simulink model "HXpump_whole"  (R2014b)
settings: Solver=FixedStepDiscrete  StartTime=0.0  StopTime=Tfinal  FixedStep=Ts  RelTol=1e-3
values from neighbouring files (symbols this model uses):
  A = wallpar(4)    [EKFdynamics.m]    (also in heatexchanger.m; heatexchangerpump.m; hxpumpcode.m = params.A; hxpumpcodesanity.m = 292.2)
  cc = coldpar(3)    [EKFdynamics.m]    (also in heatexchanger.m; heatexchangerpump.m; hxpumpcode.m = params.cc; hxpumpcodesanity.m = 1901)
  ch = hotpar(3)    [EKFdynamics.m]    (also in heatexchanger.m; heatexchangerpump.m; hxpumpcode.m = params.ch; hxpumpcodesanity.m = 2414)
  cw = wallpar(3)    [EKFdynamics.m]    (also in heatexchanger.m; heatexchangerpump.m; hxpumpcode.m = params.cw; hxpumpcodesanity.m = 578)
  filenameAsnum = uint8(filename)    [hxpumpcode.m]
  h = params.Ts    [hxpumpcode.m]    (also in hxpumpcodesanity.m = 0.1; noErrornoDelay.mat = 0.1)
  hc = coldpar(4)    [EKFdynamics.m]    (also in heatexchanger.m; heatexchangerpump.m; hxpumpcode.m = params.hc; hxpumpcodesanity.m = 24500)
  hh = hotpar(5)    [EKFdynamics.m]    (also in heatexchanger.m; heatexchangerpump.m; hxpumpcode.m = params.hh; hxpumpcodesanity.m = 23800)
  ki = 1.2    [HeatExchanger_ps.m]    (also in hxpumpcode.m = 1; hxpumpcodesanity.m; noErrornoDelay.mat = 1)
  kp = 4.995    [HeatExchanger_ps.m]    (also in hxpumpcode.m = 4; hxpumpcodesanity.m; noErrornoDelay.mat = 4)
  mdotc = input(1)    [EKFdynamics.m]    (also in heatexchanger.m; heatexchangerpump.m; hxpumpcode.m = 210.8; hxpumpcodesanity.m = 247)
  mdoth = hotpar(4)    [EKFdynamics.m]    (also in heatexchanger.m; heatexchangerpump.m; hxpumpcode.m = params.mdoth; hxpumpcodesanity.m = 350)
  PDT = [0.0475545264184 0.219864503106 0.124236222348 0.000344859251401 0.00269336621478 0 0.219864503106 2.46009324019 0.934080700726 -7.94146801374e-05 -0.000620231546177 0 ... (36 elements, 6x6)]    [noErrornoDelay.mat]
  Pref = params.Pref    [hxpumpcode.m]    (also in hxpumpcodesanity.m = 37.8; noErrornoDelay.mat = 37.8)
  rhoc = coldpar(1)    [EKFdynamics.m]    (also in heatexchanger.m; heatexchangerpump.m; hxpumpcode.m = params.rhoc; hxpumpcodesanity.m = 2020)
  rhoh = hotpar(1)    [EKFdynamics.m]    (also in heatexchanger.m; heatexchangerpump.m; hxpumpcode.m = params.rhoh; hxpumpcodesanity.m = 1940)
  rhow = wallpar(1)    [EKFdynamics.m]    (also in heatexchanger.m; heatexchangerpump.m; hxpumpcode.m = params.rhow; hxpumpcodesanity.m = 8860)
  Sv_mh = 0.05    [HeatExchanger_ps.m]    (also in hxpumpcode.m = params.Sv_mh; hxpumpcodesanity.m; noErrornoDelay.mat)
  Sv_thi = 5e-2    (= 0.05)    [HeatExchanger_ps.m]    (also in hxpumpcode.m = params.Sv_thi; hxpumpcodesanity.m; noErrornoDelay.mat)
  Sv_tho = 0.1    [HeatExchanger_ps.m]    (also in hxpumpcode.m = params.Sv_tho; hxpumpcodesanity.m; noErrornoDelay.mat)
  Sw_mh = 25    [HeatExchanger_ps.m]    (also in hxpumpcode.m = params.Sw_mh; hxpumpcodesanity.m; noErrornoDelay.mat)
  Sw_tc = 0.05    [HeatExchanger_ps.m]    (also in hxpumpcode.m = params.Sw_tc; hxpumpcodesanity.m; noErrornoDelay.mat)
  Sw_th = 25    [HeatExchanger_ps.m]    (also in hxpumpcode.m = params.Sw_th; hxpumpcodesanity.m; noErrornoDelay.mat)
  Tci = input(2)    [EKFdynamics.m]    (also in heatexchanger.m; heatexchangerpump.m; hxpumpcode.m = params.Tci; hxpumpcodesanity.m = 550)
  Thi = hotpar(6)    [EKFdynamics.m]    (also in heatexchanger.m; heatexchangerpump.m; hxpumpcode.m = params.Thi; hxpumpcodesanity.m = 700)
  Ts = delta_t    (= 0.1)    [HeatExchanger_ps.m]    (also in hxpumpcode.m = params.Ts; hxpumpcodesanity.m; noErrornoDelay.mat)
  Vc = coldpar(2)    [EKFdynamics.m]    (also in heatexchanger.m; heatexchangerpump.m; hxpumpcode.m = params.Vc; hxpumpcodesanity.m = 1.5127)
  Vh = hotpar(2)    [EKFdynamics.m]    (also in heatexchanger.m; heatexchangerpump.m; hxpumpcode.m = params.Vh; hxpumpcodesanity.m = 1.1508)
  Vw = wallpar(2)    [EKFdynamics.m]    (also in heatexchanger.m; heatexchangerpump.m; hxpumpcode.m = params.Vw; hxpumpcodesanity.m = 0.4675)
  wa = pumppar(2)    [EKFdynamics.m]    (also in hxpumpcode.m = params.wa; hxpumpcodesanity.m = 0.002; noErrornoDelay.mat = 0.002)
  wb = pumppar(3)    [EKFdynamics.m]    (also in hxpumpcode.m = params.wb; hxpumpcodesanity.m = 0.005; noErrornoDelay.mat = 0.005)
  wp = pumppar(1)    [EKFdynamics.m]    (also in heatexchangerpump.m; hxpumpcode.m = params.wp; hxpumpcodesanity.m = 0.1; noErrornoDelay.mat = 0.1)
  wref = params.wref    [hxpumpcode.m]    (also in hxpumpcodesanity.m = 0.1; noErrornoDelay.mat = 0.1)
  x0 = tempx0'    [hxpumpcode.m]    (also in hxpumpcodesanity.m = [650.29 638.4 644.3 mdoth Thi 250]; noErrornoDelay.mat = [655.2 644.46 649.75 350 700 210.8])
libraries: simulink x6, powerlib_meascontrol x3
settings Model: Creator=LabUser  LastModifiedBy=sc16user
settings DataIOCC: LimitDataPoints=off  SignalLoggingSaveFormat=ModelDataLogs
settings DebuggingCC: UnderspecifiedInitializationDetection=Classic  MergeDetectMultiDrivingBlocksExec=none  MultiTaskDSMMsg=warning  MultiTaskCondExecSysMsg=none  StateNameClashWarn=warning
settings RTWCC: IncludeERTFirstTime=on

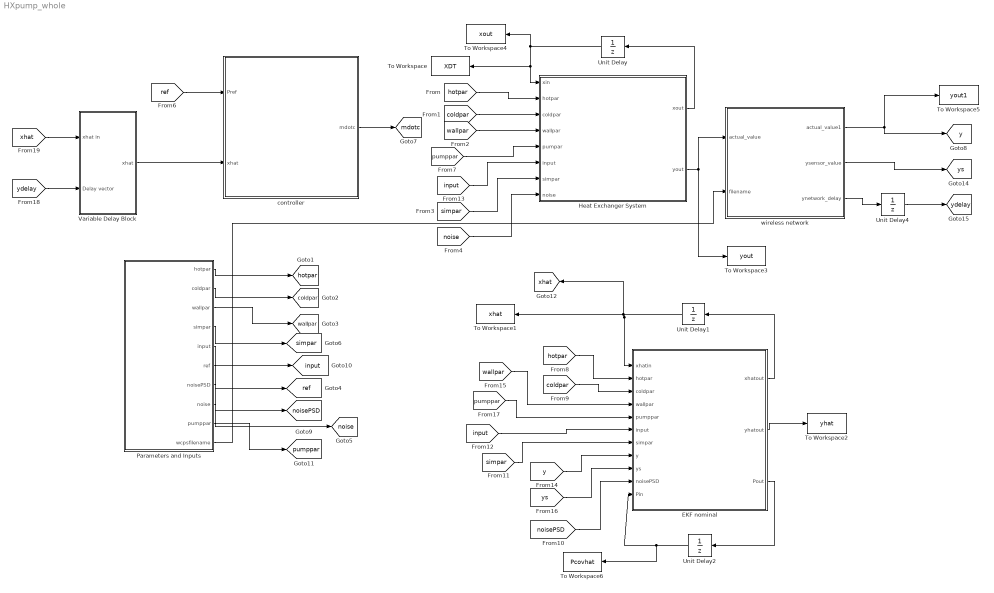
== system HXpump_whole ==
  EKF nominal : MATLAB Function  TreatAsAtomicUnit=on
  Heat Exchanger System : MATLAB Function  TreatAsAtomicUnit=on
  Parameters and Inputs : Subsystem
  To Workspace : ToWorkspace  VariableName=XDT  SampleTime=-1
  To Workspace1 : ToWorkspace  VariableName=xhat  SampleTime=-1
  To Workspace2 : ToWorkspace  VariableName=yhat  SampleTime=-1
  To Workspace3 : ToWorkspace  VariableName=yout  SampleTime=-1
  To Workspace4 : ToWorkspace  VariableName=xout  SampleTime=-1
  To Workspace5 : ToWorkspace  VariableName=yout1  SampleTime=-1
  To Workspace6 : ToWorkspace  VariableName=Pcovhat  SampleTime=-1
  Unit Delay : UnitDelay  InitialCondition=x0([1 2 3 6])  SampleTime=-1
  Unit Delay1 : UnitDelay  InitialCondition=x0  SampleTime=-1
  Unit Delay2 : UnitDelay  InitialCondition=PDT  SampleTime=-1
  Unit Delay4 : UnitDelay  InitialCondition=[0 0 0]  SampleTime=-1
  Variable Delay Block : Subsystem
  controller : Subsystem
  wireless network : MATLAB Function  TreatAsAtomicUnit=on  SystemSampleTime=0.1
  tag scope: coldpar=global, hotpar=global, input=global, mdotc=global, noise=global, noisePSD=global, pumppar=global, ref=global, simpar=global, wallpar=global, xhat=global, y=global, ydelay=global, ys=global
  wires:
  Unit Delay/1 -> To Workspace4/1, To Workspace/1, Heat Exchanger System/1(xin)
  Heat Exchanger System/1(xout) -> Unit Delay/1
  [hotpar] -> Heat Exchanger System/2(hotpar)
  [coldpar] -> Heat Exchanger System/3(coldpar)
  [wallpar] -> Heat Exchanger System/4(wallpar)
  [simpar] -> Heat Exchanger System/7(simpar)
  [noise] -> Heat Exchanger System/8(noise)
  [input] -> Heat Exchanger System/6(input)
  [ref] -> controller/1(Pref)
  Variable Delay Block/1(xhat) -> controller/2(xhat)
  controller/1(mdotc) -> [mdotc]
  [pumppar] -> Heat Exchanger System/5(pumpar)
  Parameters and Inputs/1(hotpar) -> [hotpar]
  Parameters and Inputs/2(coldpar) -> [coldpar]
  Parameters and Inputs/3(wallpar) -> [wallpar]
  Parameters and Inputs/4(simpar) -> [simpar]
  Parameters and Inputs/5(input) -> [input]
  Parameters and Inputs/6(ref) -> [ref]
  Parameters and Inputs/8(noise) -> [noise]
  Parameters and Inputs/7(noisePSD) -> [noisePSD]
  Parameters and Inputs/9(pumppar) -> [pumppar]
  [hotpar] -> EKF nominal/2(hotpar)
  [coldpar] -> EKF nominal/3(coldpar)
  [wallpar] -> EKF nominal/4(wallpar)
  [simpar] -> EKF nominal/7(simpar)
  [y] -> EKF nominal/8(y)
  [noisePSD] -> EKF nominal/10(noisePSD)
  Unit Delay1/1 -> EKF nominal/1(xhatin), To Workspace1/1, [xhat]
  EKF nominal/1(xhatout) -> Unit Delay1/1
  EKF nominal/3(Pout) -> Unit Delay2/1
  Unit Delay2/1 -> To Workspace6/1, EKF nominal/11(Pin)
  EKF nominal/2(yhatout) -> To Workspace2/1
  [input] -> EKF nominal/6(input)
  [ys] -> EKF nominal/9(ys)
  [pumppar] -> EKF nominal/5(pumppar)
  wireless network/1(actual_value1) -> [y], To Workspace5/1
  wireless network/2(ysensor_value) -> [ys]
  wireless network/3(ynetwork_delay) -> Unit Delay4/1
  Unit Delay4/1 -> [ydelay]
  Heat Exchanger System/2(yout) -> To Workspace3/1, wireless network/1(actual_value)
  [xhat] -> Variable Delay Block/1(xhat in)
  [ydelay] -> Variable Delay Block/2(Delay vector)
  Parameters and Inputs/10(wcpsfilename) -> wireless network/2(filename)

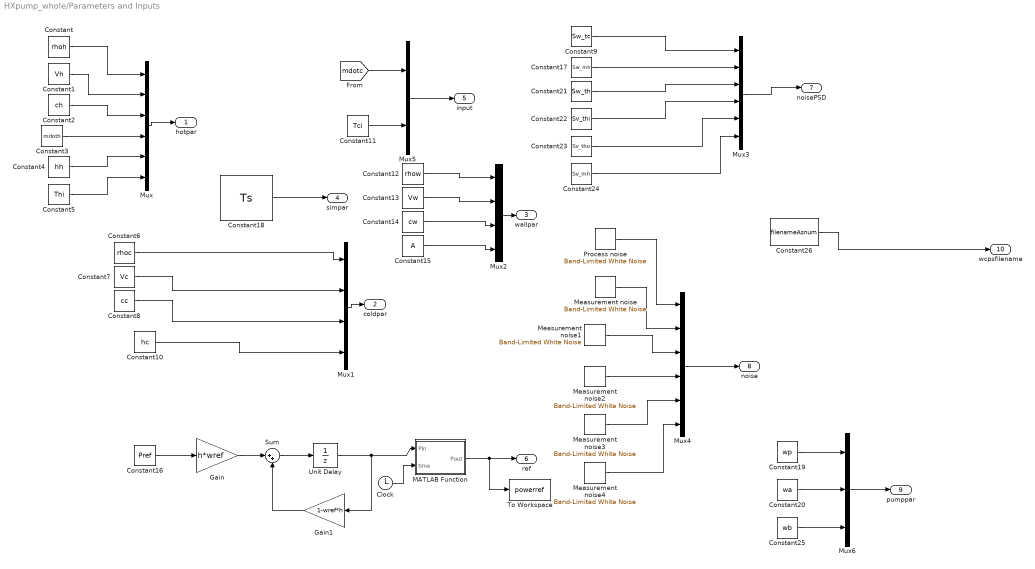
== system HXpump_whole/Parameters and Inputs ==
  Clock : Clock
  Constant : Constant  Value=rhoh  SampleTime=Ts
  Constant1 : Constant  Value=Vh  SampleTime=Ts
  Constant10 : Constant  Value=hc  SampleTime=Ts
  Constant11 : Constant  Value=Tci  SampleTime=Ts
  Constant12 : Constant  Value=rhow  SampleTime=Ts
  Constant13 : Constant  Value=Vw  SampleTime=Ts
  Constant14 : Constant  Value=cw  SampleTime=Ts
  Constant15 : Constant  Value=A  SampleTime=Ts
  Constant16 : Constant  Value=Pref  SampleTime=Ts
  Constant17 : Constant  Value=Sw_mh  SampleTime=Ts
  Constant18 : Constant  Value=Ts  SampleTime=Ts
  Constant19 : Constant  Value=wp  SampleTime=Ts
  Constant2 : Constant  Value=ch  SampleTime=Ts
  Constant20 : Constant  Value=wa  SampleTime=Ts
  Constant21 : Constant  Value=Sw_th  SampleTime=Ts
  Constant22 : Constant  Value=Sv_thi  SampleTime=Ts
  Constant23 : Constant  Value=Sv_tho  SampleTime=Ts
  Constant24 : Constant  Value=Sv_mh  SampleTime=Ts
  Constant25 : Constant  Value=wb  SampleTime=Ts
  Constant26 : Constant  Value=filenameAsnum  SampleTime=Ts
  Constant3 : Constant  Value=mdoth  SampleTime=Ts
  Constant4 : Constant  Value=hh  SampleTime=Ts
  Constant5 : Constant  Value=Thi  SampleTime=Ts
  Constant6 : Constant  Value=rhoc  SampleTime=Ts
  Constant7 : Constant  Value=Vc  SampleTime=Ts
  Constant8 : Constant  Value=cc  SampleTime=Ts
  Constant9 : Constant  Value=Sw_tc  SampleTime=Ts
  Gain : Gain  Gain=h*wref
  Gain1 : Gain  Gain=1-wref*h
  MATLAB Function : MATLAB Function  TreatAsAtomicUnit=on
  Measurement noise : simulink/Sources/Band-Limited White Noise  Cov=0  Ts=Ts  seed=[12345]
  Measurement noise1 : simulink/Sources/Band-Limited White Noise  Cov=0  Ts=Ts  seed=[23456]
  Measurement noise2 : simulink/Sources/Band-Limited White Noise  Cov=0*Ts  Ts=Ts  seed=[34567]
  Measurement noise3 : simulink/Sources/Band-Limited White Noise  Cov=0*Ts  Ts=Ts  seed=[45678]
  Measurement noise4 : simulink/Sources/Band-Limited White Noise  Cov=0*Ts  Ts=Ts  seed=[11111]
  Mux : Mux  Inputs=6
  Mux1 : Mux
  Mux2 : Mux
  Mux3 : Mux  Inputs=6
  Mux4 : Mux  Inputs=6
  Mux5 : Mux  Inputs=2
  Mux6 : Mux  Inputs=3
  Process noise : simulink/Sources/Band-Limited White Noise  Cov=0  Ts=Ts  seed=[23341]
  Sum : Sum  Inputs=|++
  To Workspace : ToWorkspace  VariableName=powerref  SampleTime=-1
  Unit Delay : UnitDelay  InitialCondition=Pref  SampleTime=-1
  hotpar : Outport
  coldpar : Outport  Port=2
  wallpar : Outport  Port=3
  simpar : Outport  Port=4
  input : Outport  Port=5
  ref : Outport  Port=6
  noisePSD : Outport  Port=7
  noise : Outport  Port=8
  pumppar : Outport  Port=9
  wcpsfilename : Outport  Port=10
  wires:
  Constant1/1 -> Mux/2
  Constant/1 -> Mux/1
  Mux/1 -> hotpar/1
  Constant2/1 -> Mux/3
  Constant6/1 -> Mux1/1
  Mux1/1 -> coldpar/1
  Constant8/1 -> Mux1/3
  Constant7/1 -> Mux1/2
  Mux2/1 -> wallpar/1
  Constant10/1 -> Mux1/4
  Constant12/1 -> Mux2/1
  Constant13/1 -> Mux2/2
  Constant14/1 -> Mux2/3
  Constant15/1 -> Mux2/4
  Constant18/1 -> simpar/1
  Constant4/1 -> Mux/5
  Mux5/1 -> input/1
  [mdotc] -> Mux5/1
  Constant11/1 -> Mux5/2
  Constant3/1 -> Mux/4
  Constant5/1 -> Mux/6
  Constant17/1 -> Mux3/2
  Constant9/1 -> Mux3/1
  Mux3/1 -> noisePSD/1
  Process noise/1 -> Mux4/1
  Measurement noise/1 -> Mux4/2
  Measurement noise1/1 -> Mux4/3
  Measurement noise2/1 -> Mux4/4
  Measurement noise3/1 -> Mux4/5
  Measurement noise4/1 -> Mux4/6
  Constant21/1 -> Mux3/3
  Constant22/1 -> Mux3/4
  Constant23/1 -> Mux3/5
  Constant24/1 -> Mux3/6
  Mux4/1 -> noise/1
  Constant16/1 -> Gain/1
  Gain/1 -> Sum/1
  Sum/1 -> Unit Delay/1
  Unit Delay/1 -> MATLAB Function/1(Pin), Gain1/1
  Gain1/1 -> Sum/2
  Constant19/1 -> Mux6/1
  Constant20/1 -> Mux6/2
  Constant25/1 -> Mux6/3
  Mux6/1 -> pumppar/1
  Clock/1 -> MATLAB Function/2(time)
  MATLAB Function/1(Pout) -> To Workspace/1, ref/1
  Constant26/1 -> wcpsfilename/1

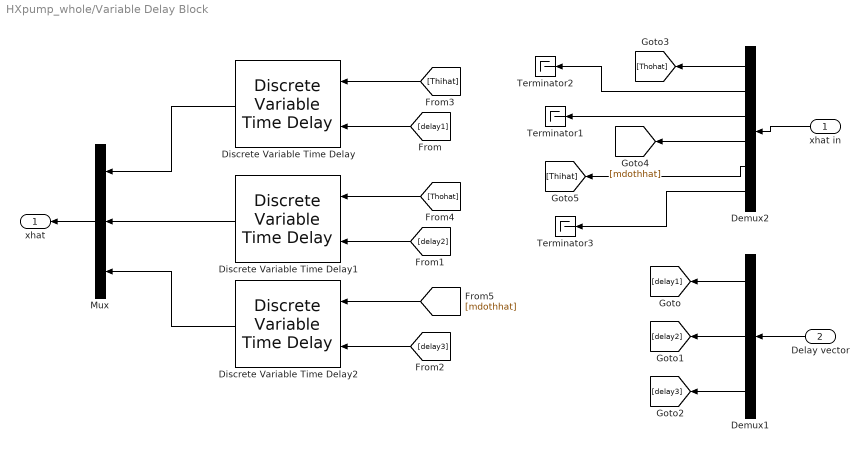
== system HXpump_whole/Variable Delay Block ==
  xhat in : Inport
  Delay vector : Inport  Port=2
  Demux1 : Demux  Outputs=3
  Demux2 : Demux  Outputs=6
  Discrete Variable Time Delay : powerlib_meascontrol/Additional Components/Discrete Variable Time Delay  MaxDelay=2  InitialValue=700  Ts=Ts  DFT=on
  Discrete Variable Time Delay1 : powerlib_meascontrol/Additional Components/Discrete Variable Time Delay  MaxDelay=2  InitialValue=650.29  Ts=Ts  DFT=on
  Discrete Variable Time Delay2 : powerlib_meascontrol/Additional Components/Discrete Variable Time Delay  MaxDelay=2  InitialValue=350  Ts=Ts  DFT=on
  Mux : Mux  Inputs=3
  Terminator1 : Terminator
  Terminator2 : Terminator
  Terminator3 : Terminator
  xhat : Outport
  wires:
  Discrete Variable Time Delay2/1 -> Mux/3
  Discrete Variable Time Delay/1 -> Mux/1
  Delay vector/1 -> Demux1/1
  Discrete Variable Time Delay1/1 -> Mux/2
  Demux1/1 -> [delay1]
  Demux1/2 -> [delay2]
  Demux1/3 -> [delay3]
  [delay1] -> Discrete Variable Time Delay/2
  [delay2] -> Discrete Variable Time Delay1/2
  [delay3] -> Discrete Variable Time Delay2/2
  [Thihat] -> Discrete Variable Time Delay/1
  [Thohat] -> Discrete Variable Time Delay1/1
  [mdothhat] -> Discrete Variable Time Delay2/1
  Mux/1 -> xhat/1
  xhat in/1 -> Demux2/1
  Demux2/1 -> [Thohat]
  Demux2/4 -> [mdothhat]
  Demux2/5 -> [Thihat]
  Demux2/3 -> Terminator1/1
  Demux2/2 -> Terminator2/1
  Demux2/6 -> Terminator3/1

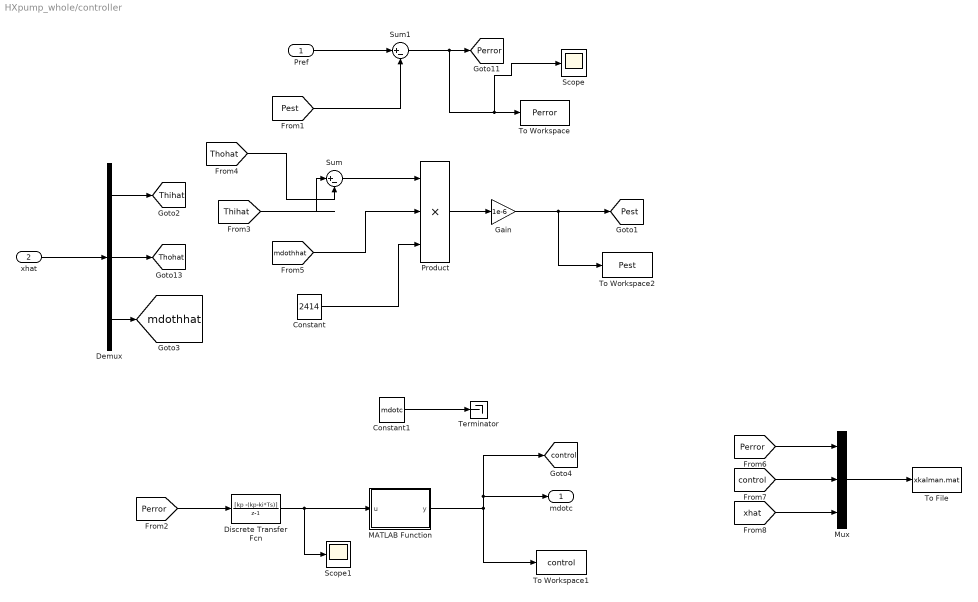
== system HXpump_whole/controller ==
  Pref : Inport
  xhat : Inport  Port=2
  Constant : Constant  Value=2414  SampleTime=Ts
  Constant1 : Constant  Value=mdotc
  Demux : Demux  Outputs=3
  Discrete Transfer Fcn : DiscreteTransferFcn  Numerator=[kp -(kp-ki*Ts)]  Denominator=[1 -1]  InitialStates=250.6/Ts  SampleTime=Ts
  Gain : Gain  Gain=1e-6
  MATLAB Function : MATLAB Function  TreatAsAtomicUnit=on
  Mux : Mux  Inputs=3
  Product : Product  Inputs=3
  Scope : Scope
  Scope1 : Scope
  Sum : Sum  Inputs=|+-
  Sum1 : Sum  Inputs=|+-
  Terminator : Terminator
  To File : ToFile  Filename=xkalman.mat  MatrixName=xkalman
  To Workspace : ToWorkspace  VariableName=Perror  SampleTime=-1
  To Workspace1 : ToWorkspace  VariableName=control  SampleTime=-1
  To Workspace2 : ToWorkspace  VariableName=Pest  SampleTime=-1
  mdotc : Outport
  tag scope: Perror=global, Pest=global, Thihat=global, Thohat=global, control=global, mdothhat=global
  wires:
  [Thohat] -> Sum/2
  [mdothhat] -> Product/2
  Sum/1 -> Product/1
  Constant/1 -> Product/3
  xhat/1 -> Demux/1
  Product/1 -> Gain/1
  Pref/1 -> Sum1/1
  Gain/1 -> To Workspace2/1, [Pest]
  [Pest] -> Sum1/2
  Sum1/1 -> To Workspace/1, Scope/1, [Perror]
  Discrete Transfer Fcn/1 -> Scope1/1, MATLAB Function/1(u)
  [Perror] -> Discrete Transfer Fcn/1
  [Thihat] -> Sum/1
  Demux/3 -> [mdothhat]
  Demux/2 -> [Thohat]
  Demux/1 -> [Thihat]
  [Perror] -> Mux/1
  [control] -> Mux/2
  Mux/1 -> To File/1
  [xhat] -> Mux/3
  Constant1/1 -> Terminator/1
  MATLAB Function/1(y) -> [control], mdotc/1, To Workspace1/1

== matlab function HXpump_whole/EKF nominal ==
  data: xhatin input; hotpar input; coldpar input; wallpar input; pumppar input; input input; simpar input; y input; ys input; noisePSD input; Pin input; xhatout output; yhatout output; Pout output
function [xhatout,yhatout,Pout] = fcn(xhatin,hotpar,coldpar,wallpar,pumppar,input,simpar,y,ys,noisePSD,Pin)
%#codegen

% simulation parameters
h = simpar(1);

% hot-leg parameters
rhoh  = hotpar(1);
Vh    = hotpar(2);
ch    = hotpar(3);
mdoth = hotpar(4);
hh    = hotpar(5);
Thi   = hotpar(6);

% cold-leg parameters
rhoc  = coldpar(1);
Vc    = coldpar(2);
cc    = coldpar(3);
hc    = coldpar(4);

% inputs
mdotc = input(1);
Tci   = input(2);

% wall parameters
rhow  = wallpar(1);
Vw    = wallpar(2);
cw    = wallpar(3);
A     = wallpar(4);

% pump and disturbance parameters
wp = pumppar(1);
wa = pumppar(2);
wb = pumppar(3);

% noisePSD
Sw_tc  = noisePSD(1);
Sw_mh  = noisePSD(2);
Sw_th  = noisePSD(3);
Sw = diag([Sw_tc Sw_mh Sw_th]);

Sv_thi = noisePSD(4);
Sv_tho = noisePSD(5);
Sv_mh  = noisePSD(6);
Sv = diag([Sv_thi Sv_tho Sv_mh]);

% fourth order Runga Kutta
c1 = 1/6;
c2 = 1/3;
c3 = 1/3;
c4 = 1/6;
a2 = 1/2;
a3 = 1/2;
a4 = 1;
b21 = 1/2;
b31 = 0;
b32 = 1/2;
b41 = 0;
b42 = 0;
b43 = 1;

K1 = EKFdynamics(xhatin,hotpar,coldpar,wallpar,pumppar,input);
K2 = EKFdynamics(xhatin+b21*K1*h,hotpar,coldpar,wallpar,pumppar,input);
K3 = EKFdynamics(xhatin+b31*K1*h+b32*K2*h,hotpar,coldpar,wallpar,pumppar,input);
K4 = EKFdynamics(xhatin+b41*K1*h+b42*K2*h+b43*K3*h,hotpar,coldpar,wallpar,pumppar,input);
slope   = c1*K1+c2*K2+c3*K3+c4*K4;

% State Matrices in Continuous-Time
ACT = [-(xhatin(4)*ch + hh*A)/(rhoh*Vh*ch) 0 hh*A/(rhoh*Vh*ch) ch*(xhatin(5) - xhatin(1))/(rhoh*Vh*ch) xhatin(4)*ch/(rhoh*Vh*ch) 0;
       0 -(mdotc*cc + hc*A)/(rhoc*Vc*cc) hc*A/(rhoc*Vc*cc) 0 0 cc*(Tci-xhatin(2))/(rhoc*Vc*cc);
       hh*A/(rhow*Vw*cw) hc*A/(rhow*Vw*cw) -(hh*A + hc*A)/(rhow*Vw*cw) 0 0 0;
       0 0 0 -wa 0 0;
       0 0 0 0 -wb 0;
       0 0 0 0 0 -wp];
BwCT = [0 0 0  ; mdotc*cc/(rhoc*Vc*cc)*Tci 0 0 ; zeros(1,3); 0 1 0;0 0 1; 0 0 0];
CCT  = [0 0 0 0 1 0; 1 0 0 0 0 0; 0 0 0 1 0 0];

% State Matrices in Discrete-Time
ADT = eye(6) + ACT*h+ACT^2*h^2/2+ACT^3*h^3/6+ACT^4*h^4/24;
BwDT = BwCT*h + ACT*BwCT*h^2/2 + 1/6*ACT^2*BwCT*h^3 + 1/24*ACT^3*BwCT*h^4;
CDT = CCT;

% State and Error Covariance Predictions
xhat = xhatin + slope*h;
Pneg = ADT*Pin*ADT' + BwDT*Sw*BwDT';

% % Correction eqautions
yhat = CDT*xhat;

if ys(2) ==1
    inov = y - yhat;
    inocov = CDT*Pneg*CDT'+Sv;
    L = Pneg*CDT'*inv(inocov);
    xhatout = xhat + L*inov;
    Pout = (eye(6)-L*CDT)*Pneg;
else
    xhatout = xhat;
    Pout = Pneg;
end

yhatout = yhat;

== matlab function HXpump_whole/Heat Exchanger System ==
  data: xin input; xout output; hotpar input; coldpar input; wallpar input; pumpar input; input input; simpar input; noise input; yout output
function [xout,yout] = fcn(xin,hotpar,coldpar,wallpar,pumpar,input,simpar,noise)
%#codegen

% simulation parameters
h = simpar(1);

% Sensor noise
v_thi = noise(4);
v_tho = noise(5);
v_mh  = noise(6);
v = [v_thi ; v_tho ; v_mh];

% hot-leg parameters
Thi   = hotpar(6);
mdoth = hotpar(4);

% fourth order Runga Kutta

c1 = 1/6;
c2 = 1/3;
c3 = 1/3;
c4 = 1/6;
a2 = 1/2;
a3 = 1/2;
a4 = 1;
b21 = 1/2;
b31 = 0;
b32 = 1/2;
b41 = 0;
b42 = 0;
b43 = 1;

%%%%% System dynamics

K1 = heatexchangerpump(xin,hotpar,coldpar,wallpar,pumpar,input,noise);
K2 = heatexchangerpump(xin+b21*K1*h,hotpar,coldpar,wallpar,pumpar,input,noise);
K3 = heatexchangerpump(xin+b31*K1*h+b32*K2*h,hotpar,coldpar,wallpar,pumpar,input,noise);
K4 = heatexchangerpump(xin+b41*K1*h+b42*K2*h+b43*K3*h,hotpar,coldpar,wallpar,pumpar,input,noise);
slope = c1*K1+c2*K2+c3*K3+c4*K4;

xout = xin + slope*h;
yout = [Thi; xin(1); mdoth] + eye(3)*v;

== matlab function HXpump_whole/wireless network ==
  data: actual_value input; actual_value1 output; ysensor_value output; ynetwork_delay output; filename input
function [actual_value1, ysensor_value, ynetwork_delay]  = Tossim_block(actual_value,filename)

% Inputs:
% ymea: measurement from structure

% Outputs:
% ymea1: measurement output
% ydelay: delay traces

persistent sensor_value % delay trace
persistent i  
persistent network_array
% count
%global ydelay_global
%global counter_global

iterations = 3001;

% allow these matlab functions to be used in Embedded Matlab block
eml.extrinsic('python');
eml.extrinsic('num2str');
eml.extrinsic('str2num');
eml.extrinsic('char');
eml.extrinsic('delay_summary');
eml.extrinsic('disp');
%eml.extrinsic('ps_aggregation');
eml.extrinsic('ps_text');
eml.extrinsic('for');
eml.extrinsic('end');
eml.extrinsic('fgets');
eml.extrinsic('fopen');

if isempty(i)
    i = 0;
    
    % read "network_error_delay.txt" file
    network_array= zeros(iterations, 6);
    
    %filename='noErrornoDelay.txt';
    
    
    %filename='/Users/wangwenchen/github/paper2_result/fault_model_1/schemeMICD_lpSample20_topoSample20/1_control_input.txt';
    
    filename=char(filename);
    
    text=fopen(filename);
    result=fgets(text);

    %network_array(1, :) = str2num(result);
    line_num=1;
    while ischar(result)
        if( line_num <=iterations)
            network_array(line_num, :) = str2num(result);
            result = fgets(text);
        else
            break;
        end

        line_num = line_num+1;

    end
    fclose(text);
    %disp(network_array);
end

%sen_num=structure.sen_num;

ysensor_value = [0 0 0]'; 
ynetwork_delay = [0 0 0]';



%call_count = 56; % number of slots + 1 (i.e., number of client calls made + 1) per TDMA schedule, +1 to have full 53 slots after %

%[resultz] = ps_aggregation(call_count);
i = i + 1;
%[resultz] = ps_text(i);
resultz=network_array(i, :);

%end_to_end_delivery_result_aggregated = sum(resultz);
%end_to_end_delivery_result_aggregated=resultz;

[sensor_value_tmp] = value_summary(resultz);
if i==1
    sensor_value_tmp=[1 1 1];
end
ysensor_value = sensor_value_tmp';

[network_delay_tmp] = network_delay_summary(resultz);
%disp(network_delay)
ynetwork_delay=network_delay_tmp';

disp('sensor_value')
disp(ysensor_value')
%disp('network delay')
%disp(ynetwork_delay')
disp('------------i------------')
disp(i)

%last_emergency_instance = ymea';
sensor_value = ysensor_value;


actual_value1 = [0 0 0]'; %3 sensors
actual_value1 = actual_value;


% for h_yg = 1:3
%     ydelay_global(h_yg, 1) = ysensor_value(h_yg, 1);
% end

disp('Plant 1, TOSSIM Uplink Block, is called');
%counter_global = counter_global + 1;

== matlab function HXpump_whole/Parameters and Inputs/MATLAB Function ==
  data: Pin input; Pout output; time input
function Pout = fcn(Pin,time)
%#codegen

ramp_inittime = 40;

% if time >= ramp_inittime
%     Pout = Pin + 4.2 / 15 * (time - ramp_inittime);
%     if Pout >= 42
%         Pout = 42;
%     else
%     end
% else
%     Pout = Pin;
% end

Pout = Pin;

== matlab function HXpump_whole/controller/MATLAB Function ==
  data: u input; y output
function y = fcn(u)
%#codegen

if u <0
    y=0;
else y=u;
end
